simulink model "SineWave"  (R2021b)
settings: Solver=VariableStepAuto  StartTime=0  StopTime=24  FixedStep=0.1  RelTol=1e-3
settings Model: Creator=jimd  LastModifiedBy=jimd

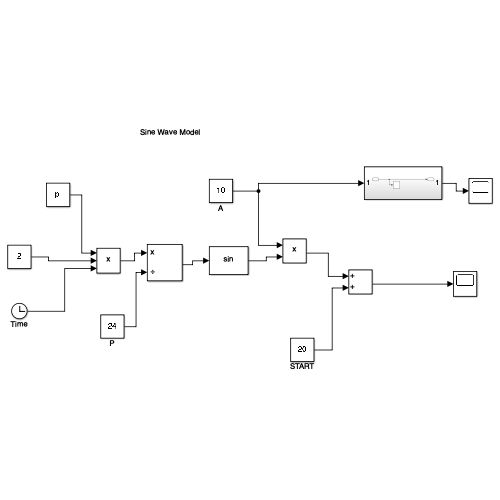
[thumbnail: Simulink's stored preview of the top-level diagram]
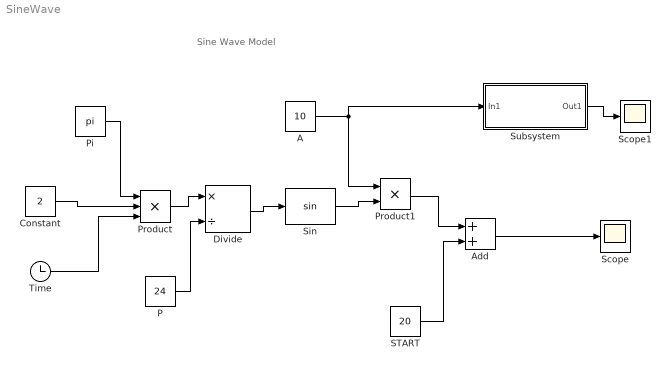
== system SineWave ==
  note: Sine Wave Model
  A : Constant  Value=10
  Add : Sum
  Constant : Constant  Value=2
  Divide : Product  Inputs=*/
  P : Constant  Value=24
  Pi : Constant  Value=pi  OutDataTypeStr=Inherit: Inherit via back propagation
  Product : Product  Inputs=3
  Product1 : Product
  START : Constant  Value=20
  Scope : Scope
  Scope1 : Scope
  Sin : Trigonometry
  Subsystem : Subsystem
  Time : Clock
  wires:
  Pi/1 -> Product/1
  Constant/1 -> Product/2
  Time/1 -> Product/3
  Product/1 -> Divide/1
  P/1 -> Divide/2
  Divide/1 -> Sin/1
  Sin/1 -> Product1/2
  A/1 -> Product1/1, Subsystem/1(In1)
  Product1/1 -> Add/1
  START/1 -> Add/2
  Add/1 -> Scope/1
  Subsystem/1(Out1) -> Scope1/1

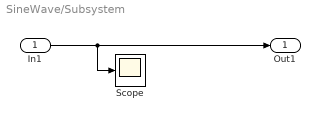
== system SineWave/Subsystem ==
  In1 : Inport
  Scope : Scope
  Out1 : Outport
  wires:
  In1/1 -> Scope/1, Out1/1
